simulink model "bpsk_sim"  (R2018b)
settings: Solver=VariableStepAuto  StartTime=0.0  StopTime=0.0  RelTol=1e-3
libraries: commrandsrc3 x1
settings Model: Creator=DSP  LastModifiedBy=DSP

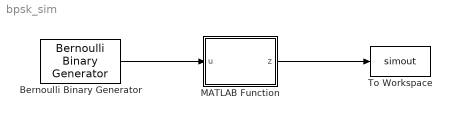
== system bpsk_sim ==
  Bernoulli Binary Generator : commrandsrc3/Bernoulli Binary Generator  ProbabilityOfZero=0.5  SeedSource=Auto  Seed=0  SampleTime=1  SamplesPerFrame=10000  OutputDataType=double  SimulateUsing=Interpreted execution
  MATLAB Function : MATLAB Function  TreatAsAtomicUnit=on
  To Workspace : ToWorkspace  VariableName=simout  SampleTime=-1
      settings: Save2DSignal=2-D array (concatenate along first dimension)
  wires:
  Bernoulli Binary Generator/1 -> MATLAB Function/1(u)
  MATLAB Function/1(z) -> To Workspace/1

== matlab function bpsk_sim/MATLAB Function ==
  data: u input; z output
function z = fcn(u)
y = zeros(length(u), 1);
for i=1:length(u)
    if u(i) == 0
        y(i) = -1;
    else
        y(i) = 1;
    end
end

awgn = randn(length(u), 1);
snrdb = 0:24;
snr = 0:24;
err = 0:24;
err_rate = 0:24;
for j = 1:length(snrdb)
    snr(j) = 10^(snrdb(j)/10);
    sigma = 1/sqrt(snr(j));
    yr = y + sigma*awgn;
    for i=1:length(yr)
        if yr(i) > 0
            yr(i) = 1;
        else
            yr(i) = 0;
        end
    end
    err(j) = sum(abs(u - yr));
    err_rate(j) = err(j)/length(u);
end


z = err_rate;
